simulink model "step2"  (R2021a)
settings: Solver=VariableStepAuto  StartTime=0.0  StopTime=10.0  RelTol=1e-3
settings Model: Creator=konsta  LastModifiedBy=konsta

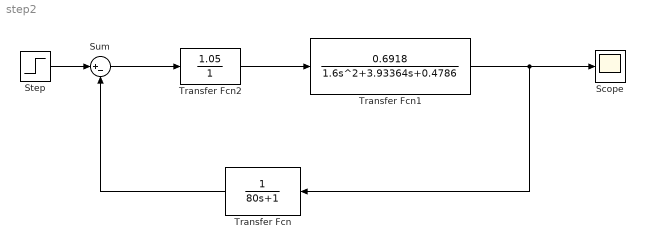
== system step2 ==
  Scope : Scope
  Step : Step  SampleTime=0
  Sum : Sum  Inputs=|+-
  Transfer Fcn : TransferFcn  Denominator=[80 1]
  Transfer Fcn1 : TransferFcn  Numerator=[0.6918]  Denominator=[1.6 3.93364 0.4786]
  Transfer Fcn2 : TransferFcn  Numerator=[1.05]  Denominator=[0 1]
  wires:
  Sum/1 -> Transfer Fcn2/1
  Transfer Fcn2/1 -> Transfer Fcn1/1
  Step/1 -> Sum/1
  Transfer Fcn/1 -> Sum/2
  Transfer Fcn1/1 -> Scope/1, Transfer Fcn/1
